simulink model "usmc2_circle"  (R2020b)
settings: Solver=VariableStepAuto  StartTime=0.0  StopTime=200  RelTol=1e-3
settings Model: Creator=Lenovo  LastModifiedBy=Lenovo

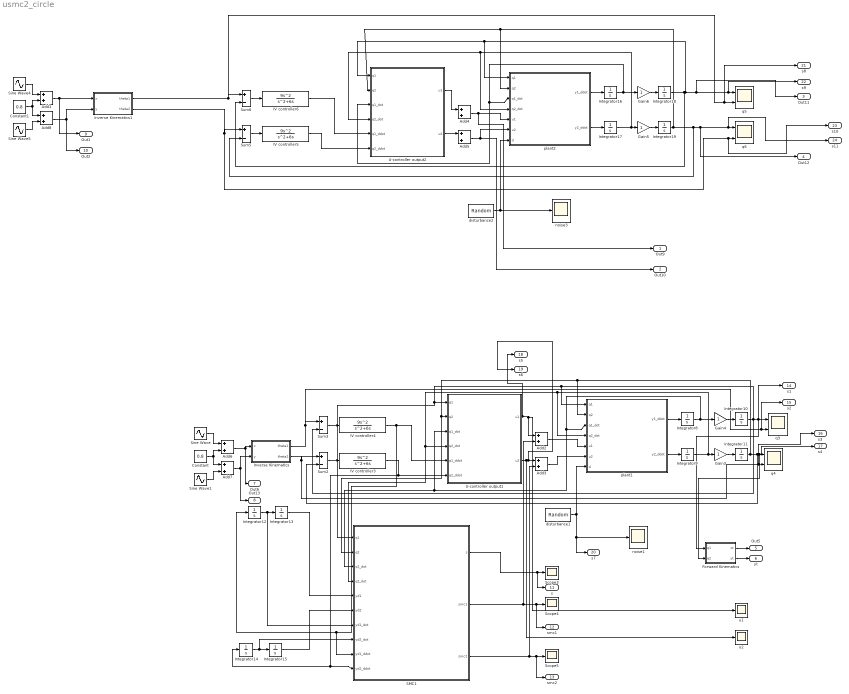
== system usmc2_circle ==
  Add{1..8} (8 alike) : Sum
  Constant : Constant  Value=0.8
  Constant1 : Constant  Value=0.8
  Forward Kinematics : MATLAB Function  TreatAsAtomicUnit=on
  Gain{3..6} (4 alike) : Gain
  IV controller{3..6} (4 alike) : TransferFcn  Numerator=[9 0 0]  Denominator=[1 6 0]
  Integrator{8..19} (12 alike) : Integrator
  Inverse Kinematics : MATLAB Function  TreatAsAtomicUnit=on
  Inverse Kinematics1 : MATLAB Function  TreatAsAtomicUnit=on
  SMC1 : MATLAB Function  TreatAsAtomicUnit=on
  Scope3 : Scope
  Scope4 : Scope
  Scope5 : Scope
  Sine Wave : Sin  Amplitude=0.4  Frequency=0.4  SampleTime=0.001
  Sine Wave1 : Sin  Amplitude=0.4  Frequency=0.4  Phase=-1.57  SampleTime=0.001
  Sine Wave4 : Sin  Amplitude=0.4  Frequency=0.4  SampleTime=0.001
  Sine Wave5 : Sin  Amplitude=0.4  Frequency=0.4  Phase=-1.57  SampleTime=0.001
  Sum{2..3,5..6} (4 alike) : Sum  Inputs=|+-
  U-controller output1 : MATLAB Function  TreatAsAtomicUnit=on
  U-controller output2 : MATLAB Function  TreatAsAtomicUnit=on
  disturbance1 : UniformRandomNumber  Minimum=-0.2  Maximum=0.2  SampleTime=0.01
  disturbance2 : UniformRandomNumber  Minimum=-0.2  Maximum=0.2  SampleTime=0.01
  noise1 : Scope
  noise3 : Scope
  plant1 : MATLAB Function  TreatAsAtomicUnit=on
  plant2 : MATLAB Function  TreatAsAtomicUnit=on
  q{3..6} (4 alike) : Scope  NumInputPorts=2
  u1 : Scope
  u2 : Scope
  Out9 : Outport  VectorParamsAs1DForOutWhenUnconnected=off
  Out10 : Outport  Port=2  VectorParamsAs1DForOutWhenUnconnected=off
  Out11 : Outport  Port=3  VectorParamsAs1DForOutWhenUnconnected=off
  Out12 : Outport  Port=4  VectorParamsAs1DForOutWhenUnconnected=off
  Out5 : Outport  Port=5
  yt : Outport  Port=6
  Out6 : Outport  Port=7
  Out13 : Outport  Port=8
  Out1 : Outport  Port=9
  Out2 : Outport  Port=10
  s : Outport  Port=11
  smc1 : Outport  Port=12
  smc2 : Outport  Port=13
  s1 : Outport  Port=14
  s2 : Outport  Port=15
  s3 : Outport  Port=16
  s4 : Outport  Port=17
  s5 : Outport  Port=18
  s6 : Outport  Port=19
  s7 : Outport  Port=20
  s8 : Outport  Port=21
  s9 : Outport  Port=22
  s10 : Outport  Port=23
  s11 : Outport  Port=24
  wires:
  Add3/1 -> plant1/6(u2)
  Integrator14/1 -> SMC1/8(yd2_dot), Integrator15/1
  IV controller4/1 -> SMC1/9(yd1_ddot), Integrator12/1, U-controller output1/5(q1_ddot)
  Sum3/1 -> IV controller4/1
  Integrator13/1 -> SMC1/5(yd1)
  Integrator15/1 -> SMC1/6(yd2)
  Add5/1 -> Out10/1, plant2/6(u2)
  Add2/1 -> plant1/5(u1)
  Integrator8/1 -> Gain4/1, SMC1/3(q1_dot), U-controller output1/3(q1_dot), plant1/3(q1_dot)
  Gain6/1 -> Integrator18/1
  Integrator19/1 -> Out12/1, s11/1, q6/1, Sum5/2, U-controller output2/2(q2), plant2/2(q2)
  plant2/1(y1_ddot) -> Integrator16/1
  Integrator16/1 -> Gain6/1, U-controller output2/3(q1_dot), plant2/3(q1_dot)
  Gain4/1 -> Integrator10/1
  IV controller3/1 -> SMC1/10(yd2_ddot), Integrator14/1, U-controller output1/6(q2_ddot)
  Add4/1 -> Out9/1, plant2/5(u1)
  Integrator9/1 -> U-controller output1/4(q2_dot), SMC1/4(q2_dot), plant1/4(q2_dot), Gain3/1
  SMC1/1(s) -> s/1, Scope3/1
  Sum5/1 -> IV controller5/1
  IV controller6/1 -> U-controller output2/5(q1_ddot)
  Sum6/1 -> IV controller6/1
  disturbance2/1 -> plant2/7(d), noise3/1
  U-controller output2/2(u2) -> Add5/1
  plant2/2(y2_ddot) -> Integrator17/1
  Gain3/1 -> Integrator11/1
  Inverse Kinematics/2(theta2) -> s3/1, q4/2, Sum2/1
  Inverse Kinematics/1(theta1) -> s2/1, q3/2, Sum3/1
  Gain5/1 -> Integrator19/1
  U-controller output1/2(u2) -> s6/1, Add3/1, u2/1
  Integrator11/1 -> s4/1, Forward Kinematics/2(q2), q4/1, Sum2/2, SMC1/2(q2), U-controller output1/2(q2), plant1/2(q2)
  SMC1/3(smc2) -> Add3/2, smc2/1, Scope5/1
  SMC1/2(smc1) -> Add2/2, smc1/1, Scope4/1
  plant1/2(y2_ddot) -> Integrator9/1
  U-controller output2/1(u1) -> Add4/1
  disturbance1/1 -> s7/1, noise1/1, plant1/7(d)
  plant1/1(y1_ddot) -> Integrator8/1
  Inverse Kinematics1/2(theta2) -> s10/1, q6/2, Sum5/1
  Integrator10/1 -> s1/1, q3/1, Forward Kinematics/1(q1), SMC1/1(q1), U-controller output1/1(q1), plant1/1(q1), Sum3/2
  Sum2/1 -> IV controller3/1
  IV controller5/1 -> U-controller output2/6(q2_ddot)
  U-controller output1/1(u1) -> s5/1, u1/1, Add2/1
  Integrator17/1 -> U-controller output2/4(q2_dot), plant2/4(q2_dot), Gain5/1
  Integrator18/1 -> Out11/1, s9/1, q5/1, U-controller output2/1(q1), plant2/1(q1), Sum6/2
  Integrator12/1 -> SMC1/7(yd1_dot), Integrator13/1
  Sine Wave/1 -> Add6/1
  Sine Wave1/1 -> Add7/2
  Forward Kinematics/1(xt) -> Out5/1
  Forward Kinematics/2(yt) -> yt/1
  Constant/1 -> Add7/1, Add6/2
  Add7/1 -> Inverse Kinematics/2(y), Out13/1
  Add6/1 -> Out6/1, Inverse Kinematics/1(x)
  Sine Wave5/1 -> Add8/2
  Add8/1 -> Out2/1, Inverse Kinematics1/2(y)
  Constant1/1 -> Add8/1, Add1/2
  Add1/1 -> Out1/1, Inverse Kinematics1/1(x)
  Sine Wave4/1 -> Add1/1
  Inverse Kinematics1/1(theta1) -> s8/1, q5/2, Sum6/1

== matlab function usmc2_circle/plant2 ==
  data: q1 input; y1_ddot output; q2 input; q1_dot input; q2_dot input; y2_ddot output; u1 input; u2 input; d input
function [y1_ddot, y2_ddot] = fcn(q1, q2, q1_dot, q2_dot, u1, u2, d)

m1 = 1; m2 = 1;
l1 = 1; l2 = 1;
g = 9.8;
c2 = cos(q2);
s2 = sin(q2);
h = -0.5*m2*l1*l2*s2;
c1 = cos(q1);
c2 = cos(q2);
c12 = cos(q1+q2);


H = [1/3*m1*l1*l1+m2*l1*l1+1/3*m2*l2*l2+m2*l1*l2*c2, 1/3*m2*l2*l2+0.5*m2*l1*l2*c2;
    1/3*m2*l2*l2+1/2*m2*l1*l2*c2, 1/3*m2*l2*l2];

C = [h*q2_dot, h*(q1_dot+q2_dot);
     -h*q1_dot, 0];
 
G = [0.5*m1*g*l1*c1+m2*g*l1*c1+0.5*m2*g*l2*c12;
     0.5*m2*g*l2*c12];

output = inv(H) * ( [u1;u2] - C * [q1_dot;q2_dot] - G - d);

%%%%%% d means disturbance
y1_ddot = output(1,1);
y2_ddot = output(2,1);

== matlab function usmc2_circle/Inverse Kinematics ==
  data: x input; theta1 output; y input; theta2 output
function [theta1,theta2]= fcn(x,y)

l1=1; l2=1;
cos2 = (x.^2 + y.^2 - l1.^2 - l2.^2)/(2*l1*l2);

theta2_ = [acos(cos2) ; -acos(cos2) ];

% first set angle
theta2 = theta2_(1);
k1 = l1+l2*cos(theta2);
k2 = l2 * sin(theta2);
theta1 = atan(y/x) - atan(k2/k1);

== matlab function usmc2_circle/Inverse Kinematics1 ==
  data: x input; theta1 output; y input; theta2 output
function [theta1,theta2]= fcn(x,y)

l1=1; l2=1;
cos2 = (x.^2 + y.^2 - l1.^2 - l2.^2)/(2*l1*l2);

theta2_ = [acos(cos2) ; -acos(cos2) ];

% first set angle
theta2 = theta2_(1);
k1 = l1+l2*cos(theta2);
k2 = l2 * sin(theta2);
theta1 = atan(y/x) - atan(k2/k1);

== matlab function usmc2_circle/SMC1 ==
  data: q1 input; s output; q2 input; q1_dot input; q2_dot input; smc1 output; yd1 input; yd2 input; yd1_dot input; yd2_dot input; yd1_ddot input; yd2_ddot input; smc2 output
function [s,smc1,smc2] = fcn(q1, q2, q1_dot, q2_dot, yd1,yd2,yd1_dot,yd2_dot,yd1_ddot,yd2_ddot)

m1 = 1; m2 = 1;
l1 = 1; l2 = 1;
g = 9.8;
c2 = cos(q2);
s2 = sin(q2);
h = -0.5*m2*l1*l2*s2;
c1 = cos(q1);
c2 = cos(q2);
c12 = cos(q1+q2);


H = [1/3*m1*l1*l1+m2*l1*l1+1/3*m2*l2*l2+m2*l1*l2*c2, 1/3*m2*l2*l2+0.5*m2*l1*l2*c2;
    1/3*m2*l2*l2+1/2*m2*l1*l2*c2, 1/3*m2*l2*l2];

C = [h*q2_dot, h*(q1_dot+q2_dot);
     -h*q1_dot, 0];
 
G = [0.5*m1*g*l1*c1+m2*g*l1*c1+0.5*m2*g*l2*c12;
     0.5*m2*g*l2*c12];

 
%%% smc
c1 = 10; c2 = 10; eita = 20;


z1 = [q1-yd1;q2-yd2];
z1_dot = [q1_dot-yd1_dot;q2_dot-yd2_dot];
z2 = c1 .* z1 + z1_dot;

%%%% sliding variable
s = z2;
sgn = s ./ (abs(s)+0.01);

%%%% control output
output = C * [q1_dot;q2_dot] + G + H * (-c1.*z1_dot+[yd1_ddot;yd2_ddot]-c2.*z2-z1) -eita.*sgn;

smc1 = output(1,1);
smc2 = output(2,1);

== matlab function usmc2_circle/U-controller output1 ==
  data: q1 input; u1 output; q2 input; q1_dot input; q2_dot input; u2 output; q1_ddot input; q2_ddot input
function [u1, u2] = fcn(q1, q2, q1_dot, q2_dot, q1_ddot, q2_ddot)

%%%%%%%%% Variables %%%%%%%%%%
m1 = 1; m2 = 1;
l1 = 1; l2 = 1;
g = 9.8;
c2 = cos(q2);
s2 = sin(q2);
h = -0.5*m2*l1*l2*s2;
c1 = cos(q1);
c2 = cos(q2);
co12 = cos(q1+q2);

y1_dot = q1_dot; y2_dot = q2_dot;
y1_ddot = q1_ddot; y2_ddot = q2_ddot;

%%%%%%%%% Matrix Calculation %%%%%%%%%%
H = [1/3*m1*l1*l1+m2*l1*l1+1/3*m2*l2*l2+m2*l1*l2*c2, 1/3*m2*l2*l2+0.5*m2*l1*l2*c2;
    1/3*m2*l2*l2+1/2*m2*l1*l2*c2, 1/3*m2*l2*l2];

C = [h*q2_dot, h*(q1_dot+q2_dot);
                      -h*q1_dot, 0];
c11 = C(1,1); c12 = C(1,2); c21 = C(2,1); c22 = C(2,2);                  


G = [0.5*m1*g*l1*c1+m2*g*l1*c1+0.5*m2*g*l2*co12;
     0.5*m2*g*l2*co12];
g1 = G(1,1); g2 = G(2,1);


M_ = inv(H);
m_11 = M_(1,1); m_12 = M_(1,2); m_21 = M_(2,1); m_22 = M_(2,2);

%%%%%%%%%% U-model output %%%%%%%%%%%
temp1 = -c11 * y1_dot - c12 * y2_dot - g1;
temp2 = -c21 * y1_dot - c22 * y2_dot - g2;

u1 = (m_22/m_12*y1_ddot-y2_ddot) / (m_22/m_12*m_11-m_21) - temp1;
u2 = (m_21/m_11*y1_ddot-y2_ddot) / (m_21/m_11*m_12-m_22) - temp2;

== matlab function usmc2_circle/plant1 ==
  data: q1 input; y1_ddot output; q2 input; q1_dot input; q2_dot input; y2_ddot output; u1 input; u2 input; d input
function [y1_ddot, y2_ddot] = fcn(q1, q2, q1_dot, q2_dot, u1, u2, d)

m1 = 1; m2 = 1;
l1 = 1; l2 = 1;
g = 9.8;
c2 = cos(q2);
s2 = sin(q2);
h = -0.5*m2*l1*l2*s2;
c1 = cos(q1);
c2 = cos(q2);
c12 = cos(q1+q2);


H = [1/3*m1*l1*l1+m2*l1*l1+1/3*m2*l2*l2+m2*l1*l2*c2, 1/3*m2*l2*l2+0.5*m2*l1*l2*c2;
    1/3*m2*l2*l2+1/2*m2*l1*l2*c2, 1/3*m2*l2*l2];

C = [h*q2_dot, h*(q1_dot+q2_dot);
     -h*q1_dot, 0];
 
G = [0.5*m1*g*l1*c1+m2*g*l1*c1+0.5*m2*g*l2*c12;
     0.5*m2*g*l2*c12];


output = inv(H) * ( [u1;u2] - C * [q1_dot;q2_dot] - G - d);

%%%%%% d means disturbance
y1_ddot = output(1,1);
y2_ddot = output(2,1);

== matlab function usmc2_circle/Forward Kinematics ==
  data: q1 input; xt output; q2 input; yt output
function [xt,yt] = fcn(q1,q2)


%% Links Lengths
l1 = 1 ;
l2 = 1 ;

%% Trigonometric abbreviations
c1 = cos(q1);
c2 = cos(q2);
c12 = cos(q1+q2);

s1= sin(q1);
s2 = sin(q2);
s12 = sin(q1+q2);

%% Tip position
% These equations are derived from the Forward Kinematic model of the 2DOF
% robot
xt = l1*c1+l2*c12 ;
yt = l1*s1+l2*s12 ;

== matlab function usmc2_circle/U-controller output2 ==
  data: q1 input; u1 output; q2 input; q1_dot input; q2_dot input; u2 output; q1_ddot input; q2_ddot input
function [u1, u2] = fcn(q1, q2, q1_dot, q2_dot, q1_ddot, q2_ddot)

%%%%%%%%% Variables %%%%%%%%%%
m1 = 1; m2 = 1;
l1 = 1; l2 = 1;
g = 9.8;
c2 = cos(q2);
s2 = sin(q2);
h = -0.5*m2*l1*l2*s2;
c1 = cos(q1);
c2 = cos(q2);
co12 = cos(q1+q2);

y1_dot = q1_dot; y2_dot = q2_dot;
y1_ddot = q1_ddot; y2_ddot = q2_ddot;

%%%%%%%%% Matrix Calculation %%%%%%%%%%
H = [1/3*m1*l1*l1+m2*l1*l1+1/3*m2*l2*l2+m2*l1*l2*c2, 1/3*m2*l2*l2+0.5*m2*l1*l2*c2;
    1/3*m2*l2*l2+1/2*m2*l1*l2*c2, 1/3*m2*l2*l2];

C = [h*q2_dot, h*(q1_dot+q2_dot);
                      -h*q1_dot, 0];
c11 = C(1,1); c12 = C(1,2); c21 = C(2,1); c22 = C(2,2);                  


G = [0.5*m1*g*l1*c1+m2*g*l1*c1+0.5*m2*g*l2*co12;
     0.5*m2*g*l2*co12];
g1 = G(1,1); g2 = G(2,1);


M_ = inv(H);
m_11 = M_(1,1); m_12 = M_(1,2); m_21 = M_(2,1); m_22 = M_(2,2);

%%%%%%%%%% U-model output %%%%%%%%%%%
temp1 = -c11 * y1_dot - c12 * y2_dot - g1;
temp2 = -c21 * y1_dot - c22 * y2_dot - g2;

u1 = (m_22/m_12*y1_ddot-y2_ddot) / (m_22/m_12*m_11-m_21) - temp1;
u2 = (m_21/m_11*y1_ddot-y2_ddot) / (m_21/m_11*m_12-m_22) - temp2;
